simulink model "GPS32"  (R2020b)
settings: Solver=FixedStepAuto  StartTime=0.0  StopTime=inf  FixedStep=0.01  RelTol=1e-3  EnableMultiTasking=on
model workspace (MAT data in the model file):
  Ts = 0.01
values from neighbouring files (symbols this model uses):
  den_lpf_d = den_lpf20    [Mainframe_init.m]    (also in load_autopilot.m)
  num_lpf_d = num_lpf20    [Mainframe_init.m]    (also in load_autopilot.m)
undefined symbols (not defined in the file or in its folder): Autopilot, AUX, dev, DiscIntNeverNeededParam, h_bkpts_m, HIL_Data, Ki_phi_vec, Kp_p_vec, Kp_phi_vec, Main, pwm_output0, pwm_output1, Tr4r3, unc_fin_def_pitch, unc_fin_def_roll, unc_fin_def_yaw, V_bkpts_mps, x, y, z
libraries: simulink_extras x11, px4uORBlib x6, px4Sensorslib x3, px4lib x3, simulink x1, sharedtransform x1
settings Model: SimulationMode=external  ExtModeTrigDuration=10  Creator=WrySi  LastModifiedBy=sasson
settings SolverCC: PositivePriorityOrder=on
settings OptimizationCC: EnhancedBackFolding=on  PassReuseOutputArgsAs=Individual arguments  ZeroExternalMemoryAtStartup=off  ZeroInternalMemoryAtStartup=off  MaxStackSize=64  OptimizeBlockOrder=speed  DifferentSizesBufferReuse=on  OptimizationCustomize=off  EfficientTunableParamExpr=on
settings DebuggingCC: MultiTaskRateTransMsg=warning  ParameterOverflowMsg=none  ParameterTunabilityLossMsg=error  SymbolicDimsDataTypeCodeGenerationDiagnostic=none
settings HardwareCC: ProdBitPerPointer=32  ProdBitPerSizeT=32  ProdBitPerPtrDiffT=32  ProdLargestAtomicInteger=Long  ProdLargestAtomicFloat=Double  ProdWordSize=32  ProdLongLongMode=on  ProdHWDeviceType=ARM Compatible->ARM Cortex
settings SFSimCC: MATLABDynamicMemAlloc=off  SimTargetLang=C++
settings RTWCC: Description=Embedded Coder  SystemTargetFile=ert.tlc  HardwareBoard=PX4 Pixhawk 2.1 (Cube)  TLCOptions="-aInlineSetEventsForThisBaseRateFcn=TLC_FALSE -aSuppressMultiTaskScheduler=TLC_FALSE  -aRateBasedStepFcn=0"  TemplateMakefile=ert_default_tmf  GenerateReport=on  Toolchain=GNU Tools for PX4 Autopilots  IncludeHyperlinkInReport=on  LaunchReport=on  TargetLang=C++  GenerateTraceInfo=on  GenerateTraceReport=on  GenerateTraceReportSl=on  GenerateTraceReportSf=on  GenerateTraceReportEml=on
settings CodeAppCC: ForceParamTrailComments=on  IgnoreCustomStorageClasses=off  OperatorAnnotations=on  SimulinkDataObjDesc=on  SFDataObjDesc=on  InsertBlockDesc=on
settings ERTTargetCC: SupportContinuousTime=on  ExtMode=on  ExtModeMexArgs='127.0.0.1' 1 17725

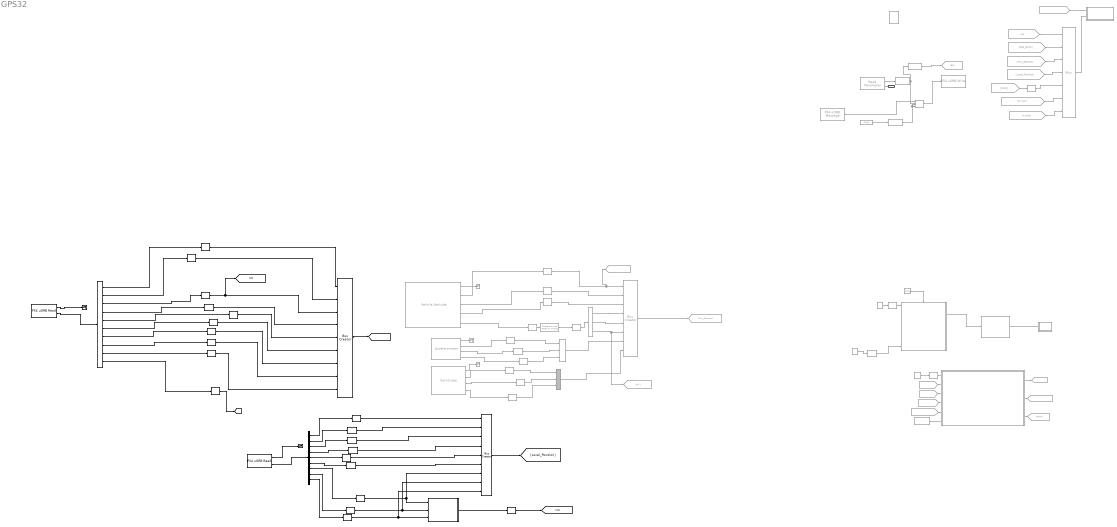
== system GPS32 ==
  note: IMU SENSORS
  note: Debag and Sound
  note: Buzzer
  note: Debag and Sound
  100 Hz : DiscretePulseGenerator  Commented=on  PulseType=Time based  Period=0.01  PulseWidth=50
  Accelerometer : px4Sensorslib/Accelerometer  Commented=on  uorbTimeStamp=off  BlockingMode=off  BlockTimeout=1e-3  sampleTime=Ts
      settings: SourceProductBaseCode=PX4AUTOPILOTS
  Bus Assignment1 : BusAssignment  Commented=on  AssignedSignals=x,z,y
  Bus Creator1 : BusCreator  Inputs=9
  Bus Creator2 : BusCreator  Inputs=9
  Bus Creator6 : BusCreator  Commented=on  Inputs=8
  Bus Creator7 : BusCreator  Commented=on  Inputs=3
  Bus Creator8 : BusCreator  Commented=on  Inputs=3
  Bus Selector1 : BusSelector  OutputSignals=ax,ay,az,z,x,y,vx,vy,vz
  Bus Selector2 : BusSelector  OutputSignals=lat,lon,alt,fix_type,satellites_used,vel_m_s,vel_n_m_s,vel_e_m_s,vel_d_m_s,timestamp
  Cast To Boolean2 : DataTypeConversion  Commented=on  OutDataTypeStr=boolean
  Cast To Double{1,3..9,11,17,21,24..31,33} (20 alike) : DataTypeConversion  OutDataTypeStr=double
  Cast To Double{2,10,12..16,18..20,22..23,32,34..35} (15 alike) : DataTypeConversion  Commented=on  OutDataTypeStr=double
  Constant : Constant  Commented=on  Value=0  SampleTime=Ts
  Constant1 : Constant  Commented=on  Value=0  SampleTime=Ts
  Constant2 : Constant  Commented=on  Value=0  SampleTime=Ts
  Data Type Conversion1 : DataTypeConversion  Commented=on  OutDataTypeStr=single
  Data Type Conversion3 : DataTypeConversion  Commented=on  OutDataTypeStr=single
  Demux2 : Demux  Commented=on  Outputs=3
  Digital Clock2 : DigitalClock  Commented=on
  Fin Allocation : Subsystem  Commented=on
  From : From  Commented=on  GotoTag=Vel
  From1 : From  Commented=on  GotoTag=Alt
  From11 : From  Commented=on  GotoTag=Local_Position
  From14 : From  Commented=on  GotoTag=EN
  From16 : From  Commented=on  GotoTag=Imu_Sensors
  From17 : From  Commented=on  GotoTag=GPS_DATA
  From18 : From  Commented=on  GotoTag=PWM
  From2 : From  Commented=on  GotoTag=P
  From3 : From  Commented=on  GotoTag=Phi
  From4 : From  Commented=on
  From7 : From  Commented=on  GotoTag=P_Filter
  From9 : From  Commented=on  GotoTag=Phi_Con
  Goto10 : Goto  Commented=on  GotoTag=EN
  Goto2 : Goto  Commented=on  GotoTag=P
  Goto3 : Goto  Commented=on  GotoTag=Phi
  Goto5 : Goto  Commented=on  GotoTag=Imu_Sensors
  Goto7 : Goto  Commented=on  GotoTag=PWM
  Goto8 : Goto  Commented=on  GotoTag=P_Filter
  Goto9 : Goto  Commented=on  GotoTag=Phi_Con
  Gyroscope : px4Sensorslib/Gyroscope  Commented=on  uorbTimeStamp=off  BlockingMode=off  BlockTimeout=1e-3  sampleTime=Ts
      settings: SourceProductBaseCode=PX4AUTOPILOTS
  Heartbeat Counter : Subsystem  Commented=on
  MATLAB Function : MATLAB Function  TreatAsAtomicUnit=on
  Mux : Mux  Commented=on  Inputs=7
  PX4 SD Card Logger3 : Subsystem  Commented=on  mask(PX4 SD Card Logger){logfile=/fs/microsd/log, logfilename=pwm, cacheflag=off, numRecs=100000000000000}
      mask prompts: logfile "Log Folder"; logfilename "Log File Name"; cacheflag "Cache in Memory"; numRecs "Maximum Record Count"
      mask help:
      | Log data to a specified file on the SD card
      |
      | The block accepts two inputs, enable and data. The incoming data is logged into the SD card when the enable signal is high and the number of data points logged is less than the Maximum Record Count specified.
      |
      | The specified folder should be present in the SD card for logging.
      |
      | If Cache in Memory is unchecked, the data is written to the SD card at every timestep.  If Cache in Memory is checked, data is cached in the memory and is written to SD card only when enable goes low or when the number of data points logged reaches the Maximum Record Count specified.
      mask init:
      | logname=uint8([logfile,'/',logfilename]);
      mask Help: eval('codertarget.internal.helpView(''px4'',''px4sdcardexample'')');
      mask Display:
      | fprintf([get_param(gcb,'logfile'),'/',get_param(gcb,'logfilename')])
      | port_label('input',1,'en')
      | port_label('input',2,'data')
  PX4 uORB Message : px4uORBlib/PX4 uORB Message  Commented=on  uORBTopic=debug_vect  SampleTime=1  selectInstance=debug_vect
      settings: SourceProductBaseCode=PX4AUTOPILOTS
  PX4 uORB Read1 : px4uORBlib/PX4 uORB Read  uORBTopic=vehicle_local_position  selectInstance=vehicle_local_position  SampleTime=Ts  BlockingMode=off  BlockTimeout=1e-3
      settings: SourceProductBaseCode=PX4AUTOPILOTS
  PX4 uORB Read2 : px4uORBlib/PX4 uORB Read  uORBTopic=vehicle_gps_position  selectInstance=vehicle_gps_position  SampleTime=Ts  BlockingMode=off  BlockTimeout=1e-3
      settings: SourceProductBaseCode=PX4AUTOPILOTS
  PX4 uORB Write : px4uORBlib/PX4 uORB Write  Commented=on  uORBTopic=debug_vect  selectInstance=debug_vect  MessageQueueLen=1
      settings: SourceProductBaseCode=PX4AUTOPILOTS
  Phi Controller : Subsystem  Commented=on
  PixBlock2 : Subsystem  Commented=on
  Quaternions to Rotation Angles2 : sharedtransform/Quaternions to Rotation Angles  Commented=on  rotationOrder=ZYX  aMode=aMode
      settings: SourceProductBaseCode=AE,PW,DR,MT,UV,VE
  Read Parameter1 : px4lib/Read Parameter  Commented=on  ParameterName=SD_save_flag  DataType=INT32  SampleTime=1
      settings: SourceProductBaseCode=PX4AUTOPILOTS
  Servos : Subsystem  Commented=on
  Subsystem2 : Subsystem  Commented=on
  Terminator1 : Terminator
  Terminator3 : Terminator
  Terminator7 : Terminator  Commented=on
  Terminator8 : Terminator  Commented=on
  Terminator9 : Terminator  Commented=on
  Vehicle Attitude : px4Sensorslib/Vehicle Attitude  Commented=on  rollRate=on  pitchRate=on  yawRate=on  quaternion=on  uorbTimeStamp=off  BlockingMode=off  BlockTimeout=0.001  sampleTime=Ts
      settings: SourceProductBaseCode=PX4AUTOPILOTS
  Out1 : Outport
  wires:
  Bus Selector2/9 -> Cast To Double11/1  "<vel_d_m_s>"
  Bus Selector2/6 -> Cast To Double7/1  "<vel_m_s>"
  Gyroscope/4 -> Cast To Double18/1  "gyroZ"
  Accelerometer/4 -> Cast To Double10/1  "accZ"
  Accelerometer/1 -> Terminator7/1
  Cast To Double2/1 -> Quaternions to Rotation Angles2/1
  Gyroscope/3 -> Cast To Double19/1  "gyroY"
  Vehicle Attitude/5 -> Cast To Double2/1
  Bus Creator7/1 -> Bus Creator6/7  "accelerometer"
  Gyroscope/1 -> Terminator9/1
  Gyroscope/2 -> Cast To Double20/1  "gyroX"
  Bus Selector2/3 -> Cast To Double4/1  "<alt>"
  Accelerometer/3 -> Cast To Double12/1  "accY"
  Accelerometer/2 -> Cast To Double13/1  "accX"
  Bus Creator8/1 -> Bus Creator6/8  "gyro"
  Vehicle Attitude/2 -> Cast To Double16/1  "p"
  Vehicle Attitude/3 -> Cast To Double15/1  "q"
  Quaternions to Rotation Angles2/1 -> Cast To Double22/1  "euler from PX conj"
  Vehicle Attitude/4 -> Cast To Double14/1  "r"
  Bus Selector2/7 -> Cast To Double8/1  "<vel_n_m_s>"
  PX4 uORB Read2/2 -> Bus Selector2/1
  Bus Selector2/8 -> Cast To Double9/1  "<vel_e_m_s>"
  Bus Selector2/1 -> Cast To Double1/1  "<lat>"
  Bus Selector2/4 -> Cast To Double5/1  "<fix_type>"
  Bus Selector2/5 -> Cast To Double6/1  "<satellites_used>"
  Vehicle Attitude/1 -> Terminator8/1
  Bus Selector2/2 -> Cast To Double3/1  "<lon>"
  Cast To Double1/1 -> Bus Creator2/1
  Cast To Double3/1 -> Bus Creator2/2
  Cast To Double4/1 -> Bus Creator2/3, [Alt]
  Cast To Double5/1 -> Bus Creator2/4
  Cast To Double6/1 -> Bus Creator2/5
  Cast To Double7/1 -> Bus Creator2/6
  Cast To Double8/1 -> Bus Creator2/7
  Cast To Double9/1 -> Bus Creator2/8
  Cast To Double11/1 -> Bus Creator2/9
  Cast To Double16/1 -> Bus Creator6/1, Goto2/1
  Cast To Double15/1 -> Bus Creator6/2
  Cast To Double14/1 -> Bus Creator6/3
  Cast To Double12/1 -> Bus Creator7/2
  Cast To Double10/1 -> Bus Creator7/3
  Cast To Double13/1 -> Bus Creator7/1
  Cast To Double20/1 -> Bus Creator8/1
  Cast To Double19/1 -> Bus Creator8/2
  Cast To Double18/1 -> Bus Creator8/3
  PX4 uORB Read2/1 -> Terminator1/1
  PX4 uORB Read1/2 -> Bus Selector1/1
  Bus Selector1/1 -> Cast To Double17/1  "<ax>"
  Bus Selector1/2 -> Cast To Double24/1  "<ay>"
  PX4 uORB Read1/1 -> Terminator3/1
  Bus Selector1/3 -> Cast To Double25/1  "<az>"
  Bus Selector1/4 -> Cast To Double26/1  "<z>"
  Bus Selector1/5 -> Cast To Double27/1  "<x>"
  Bus Selector1/6 -> Cast To Double28/1  "<y>"
  Cast To Double22/1 -> Demux2/1
  Cast To Double26/1 -> Bus Creator1/4
  Cast To Double27/1 -> Bus Creator1/5
  Cast To Double28/1 -> Bus Creator1/6
  Cast To Double25/1 -> Bus Creator1/3
  Cast To Double24/1 -> Bus Creator1/2
  Bus Assignment1/1 -> PX4 uORB Write/1
  Data Type Conversion1/1 -> Bus Assignment1/3, Bus Assignment1/4
  PX4 uORB Message/1 -> Bus Assignment1/1
  Read Parameter1/1 -> Data Type Conversion3/1
  Read Parameter1/2 -> Out1/1
  Digital Clock2/1 -> Data Type Conversion1/1
  Data Type Conversion3/1 -> Bus Assignment1/2, Cast To Boolean2/1
  Cast To Double29/1 -> Bus Creator1/7, MATLAB Function/1(vx)
  Cast To Double31/1 -> Bus Creator1/9, MATLAB Function/3(vz)
  Bus Selector1/8 -> Cast To Double30/1  "<vy>"
  Cast To Double30/1 -> Bus Creator1/8, MATLAB Function/2(vy)
  Bus Selector1/7 -> Cast To Double29/1  "<vx>"
  Bus Selector1/9 -> Cast To Double31/1  "<vz>"
  MATLAB Function/1(y) -> Cast To Double33/1
  Cast To Double23/1 -> Phi Controller/1(phi_cmd_rad)
  Constant/1 -> Cast To Double23/1
  Demux2/3 -> Goto3/1, Bus Creator6/6  "phi"
  Demux2/2 -> Bus Creator6/5  "theta"
  Demux2/1 -> Bus Creator6/4  "psi"
  Bus Creator6/1 -> Goto5/1
  Bus Creator1/1 -> [Local_Position]
  Cast To Double17/1 -> Bus Creator1/1
  Bus Creator2/1 -> [GPS_DATA]
  Cast To Double33/1 -> [Vel]
  Cast To Boolean2/1 -> Goto10/1
  From14/1 -> PX4 SD Card Logger3/1(En)
  Bus Selector2/10 -> Cast To Double21/1  "<timestamp>"
  Cast To Double21/1 -> [A]
  100 Hz/1 -> Phi Controller/Trigger
  Constant1/1 -> Cast To Double32/1
  Phi Controller/1(dela_cmd_rad) -> Fin Allocation/1(Input)  "Phi_Cmd_rad"
  Fin Allocation/1(siB_cmd) -> Servos/1(Fin Cmd)
  Cast To Double32/1 -> Phi Controller/6(integrators_active)
  From17/1 -> Mux/2
  From16/1 -> Mux/3
  From11/1 -> Mux/4
  From9/1 -> Mux/6
  From7/1 -> Mux/7
  Mux/1 -> PX4 SD Card Logger3/2(Data)
  From18/1 -> Cast To Double35/1
  Cast To Double35/1 -> Mux/5
  From4/1 -> Mux/1
  Heartbeat Counter/1(Out1) -> PixBlock2/6(Heartbeat)  "send"
  Cast To Double34/1 -> PixBlock2/1(Phi_cmd)
  Constant2/1 -> Cast To Double34/1
  From2/1 -> PixBlock2/2(P_rms)
  From1/1 -> PixBlock2/3(Alt)
  From/1 -> PixBlock2/4(Velocity)
  From3/1 -> PixBlock2/5(Phi)
  PixBlock2/2(Fin_cmd) -> Goto9/1
  PixBlock2/3(PWM) -> Goto7/1
  PixBlock2/1(P_filter) -> Goto8/1

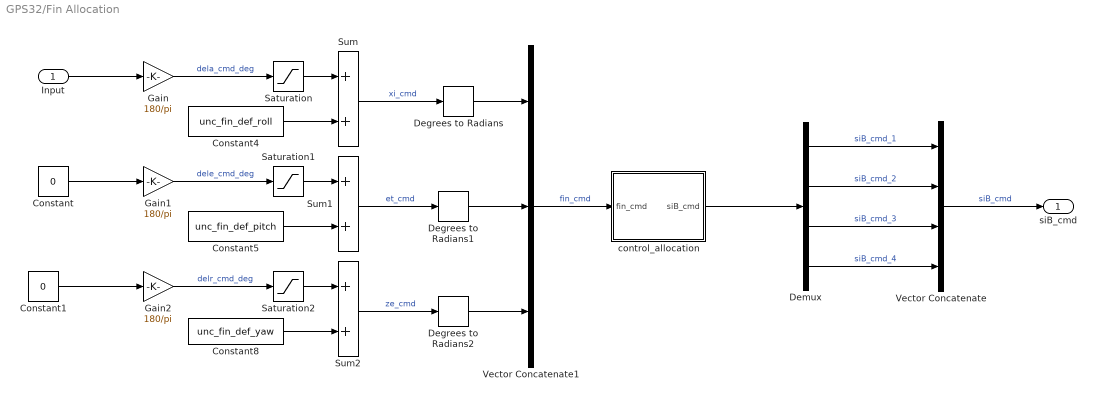
== system GPS32/Fin Allocation ==
  Input : Inport
  Constant : Constant  Value=0
  Constant1 : Constant  Value=0
  Constant4 : Constant  Value=unc_fin_def_roll
  Constant5 : Constant  Value=unc_fin_def_pitch
  Constant8 : Constant  Value=unc_fin_def_yaw
  Degrees to Radians : simulink_extras/Transformations/Degrees to Radians
  Degrees to Radians1 : simulink_extras/Transformations/Degrees to Radians
  Degrees to Radians2 : simulink_extras/Transformations/Degrees to Radians
  Demux : Demux
  Gain : Gain  Gain=180/pi
      settings: AttributesFormatString=%<Gain>
  Gain1 : Gain  Gain=180/pi
      settings: AttributesFormatString=%<Gain>
  Gain2 : Gain  Gain=180/pi
      settings: AttributesFormatString=%<Gain>
  Saturation : Saturate  UpperLimit=20  LowerLimit=-20
  Saturation1 : Saturate  UpperLimit=20  LowerLimit=-20
  Saturation2 : Saturate  UpperLimit=20  LowerLimit=-20
  Sum : Sum
  Sum1 : Sum
  Sum2 : Sum
  Vector Concatenate : Concatenate  NumInputs=4
  Vector Concatenate1 : Concatenate  NumInputs=3
  control_allocation : Subsystem
  siB_cmd : Outport  VectorParamsAs1DForOutWhenUnconnected=off
  wires:
  Constant5/1 -> Sum1/2
  Gain2/1 -> Saturation2/1  "delr_cmd_deg"
  Saturation2/1 -> Sum2/1
  Constant8/1 -> Sum2/2
  Sum2/1 -> Degrees to Radians2/1  "ze_cmd"
  Demux/3 -> Vector Concatenate/3  "siB_cmd_3"
  Constant1/1 -> Gain2/1
  Saturation/1 -> Sum/1
  Gain1/1 -> Saturation1/1  "dele_cmd_deg"
  Sum1/1 -> Degrees to Radians1/1  "et_cmd"
  Degrees to Radians/1 -> Vector Concatenate1/1
  Degrees to Radians1/1 -> Vector Concatenate1/2
  Gain/1 -> Saturation/1  "dela_cmd_deg"
  Input/1 -> Gain/1
  Degrees to Radians2/1 -> Vector Concatenate1/3
  Demux/2 -> Vector Concatenate/2  "siB_cmd_2"
  Constant4/1 -> Sum/2
  Vector Concatenate/1 -> siB_cmd/1  "siB_cmd"
  Constant/1 -> Gain1/1
  Sum/1 -> Degrees to Radians/1  "xi_cmd"
  Saturation1/1 -> Sum1/1
  Vector Concatenate1/1 -> control_allocation/1(fin_cmd)  "fin_cmd"
  Demux/1 -> Vector Concatenate/1  "siB_cmd_1"
  control_allocation/1(siB_cmd) -> Demux/1
  Demux/4 -> Vector Concatenate/4  "siB_cmd_4"

== system GPS32/Heartbeat Counter ==
  note: Starting the heartbeat at negative values prevents unwanted FCC behaviour on startup
  Cast To Double14 : DataTypeConversion  OutDataTypeStr=single
  Heartbeat : simulink/Sources/Counter Free-Running  NumBits=16  tsamp=-1
  Subtract : Sum  Inputs=+-
  Zero : Constant  Value=1000  OutDataTypeStr=Inherit: Inherit via back propagation
  Out1 : Outport
  wires:
  Heartbeat/1 -> Cast To Double14/1
  Zero/1 -> Subtract/2
  Cast To Double14/1 -> Subtract/1  "send"
  Subtract/1 -> Out1/1

== system GPS32/PX4 SD Card Logger3 ==
  En : Inport
  Data : Inport  Port=2
  SDCard_logger : MATLAB Function  TreatAsAtomicUnit=on
  Signal Specification : SignalSpecification  OutDataTypeStr=boolean
  wires:
  Data/1 -> SDCard_logger/2(data)
  En/1 -> Signal Specification/1
  Signal Specification/1 -> SDCard_logger/1(en)

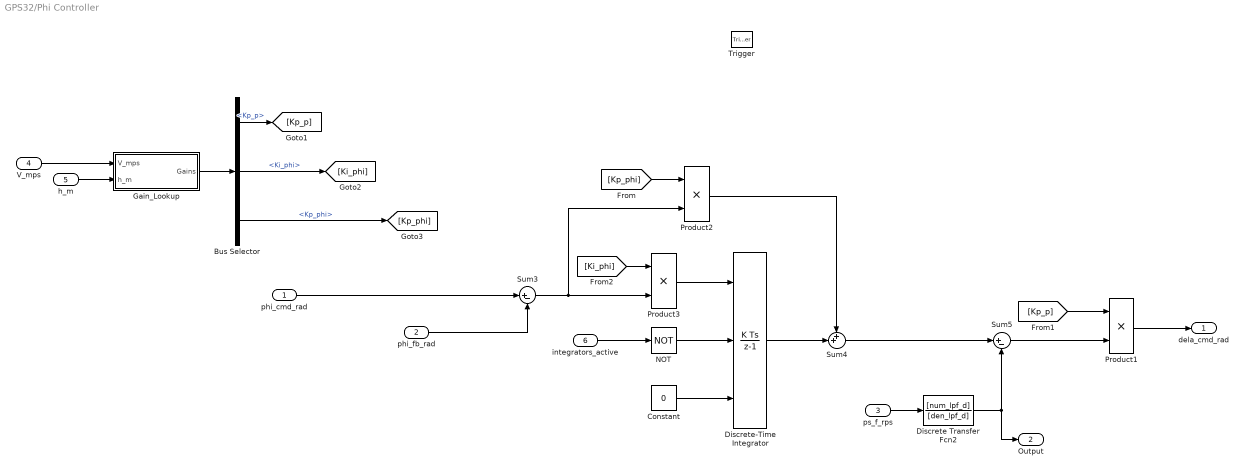
== system GPS32/Phi Controller ==
  phi_cmd_rad : Inport
  phi_fb_rad : Inport  Port=2
  ps_f_rps : Inport  Port=3
  V_mps : Inport  Port=4
  h_m : Inport  Port=5
  integrators_active : Inport  Port=6
  Trigger : TriggerPort  VariantControl=Variant  PortDimensions=1
  Bus Selector : BusSelector  OutputSignals=Kp_p,Ki_phi,Kp_phi
  Constant : Constant  Value=0  SampleTime=-1
  Discrete Transfer Fcn2 : DiscreteTransferFcn  Numerator=[num_lpf_d]  Denominator=[den_lpf_d]
  Discrete-Time Integrator : DiscreteIntegrator  ExternalReset=level  InitialConditionSource=external  SampleTime=-1  ICPrevOutput=DiscIntNeverNeededParam  ICPrevScaledInput=DiscIntNeverNeededParam
  Gain_Lookup : Subsystem
  NOT : Logic  Operator=NOT  AllPortsSameDT=off  OutDataTypeStr=boolean
  Product1 : Product
  Product2 : Product
  Product3 : Product
  Sum3 : Sum  Inputs=|+-
  Sum4 : Sum  Inputs=++|
  Sum5 : Sum  Inputs=|+-
  dela_cmd_rad : Outport
  Output : Outport  Port=2
  wires:
  Discrete-Time Integrator/1 -> Sum4/2
  NOT/1 -> Discrete-Time Integrator/2
  Bus Selector/2 -> [Ki_phi]  "<Ki_phi>"
  Product1/1 -> dela_cmd_rad/1
  ps_f_rps/1 -> Discrete Transfer Fcn2/1
  [Kp_phi] -> Product2/1
  h_m/1 -> Gain_Lookup/2(h_m)
  V_mps/1 -> Gain_Lookup/1(V_mps)
  integrators_active/1 -> NOT/1
  Constant/1 -> Discrete-Time Integrator/3
  [Kp_p] -> Product1/1
  Sum5/1 -> Product1/2
  phi_cmd_rad/1 -> Sum3/1
  Sum4/1 -> Sum5/1
  Gain_Lookup/1(Gains) -> Bus Selector/1
  Product3/1 -> Discrete-Time Integrator/1
  Bus Selector/1 -> [Kp_p]  "<Kp_p>"
  phi_fb_rad/1 -> Sum3/2
  Bus Selector/3 -> [Kp_phi]  "<Kp_phi>"
  [Ki_phi] -> Product3/1
  Product2/1 -> Sum4/1
  Sum3/1 -> Product3/2, Product2/2
  Discrete Transfer Fcn2/1 -> Output/1, Sum5/2

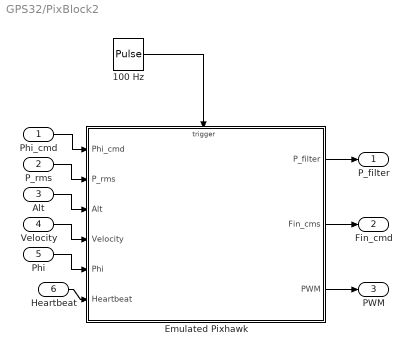
== system GPS32/PixBlock2 ==
  Phi_cmd : Inport
  P_rms : Inport  Port=2
  Alt : Inport  Port=3
  Velocity : Inport  Port=4
  Phi : Inport  Port=5
  Heartbeat : Inport  Port=6
  100 Hz : DiscretePulseGenerator  PulseType=Time based  Period=0.01  PulseWidth=50
  Emulated Pixhawk : Subsystem
  P_filter : Outport
  Fin_cmd : Outport  Port=2
  PWM : Outport  Port=3
  wires:
  100 Hz/1 -> Emulated Pixhawk/Trigger
  Emulated Pixhawk/1(P_filter) -> P_filter/1
  Phi_cmd/1 -> Emulated Pixhawk/1(Phi_cmd)
  P_rms/1 -> Emulated Pixhawk/2(P_rms)
  Phi/1 -> Emulated Pixhawk/5(Phi)
  Velocity/1 -> Emulated Pixhawk/4(Velocity)
  Alt/1 -> Emulated Pixhawk/3(Alt)
  Emulated Pixhawk/2(Fin_cms) -> Fin_cmd/1
  Heartbeat/1 -> Emulated Pixhawk/6(Heartbeat)
  Emulated Pixhawk/3(PWM) -> PWM/1

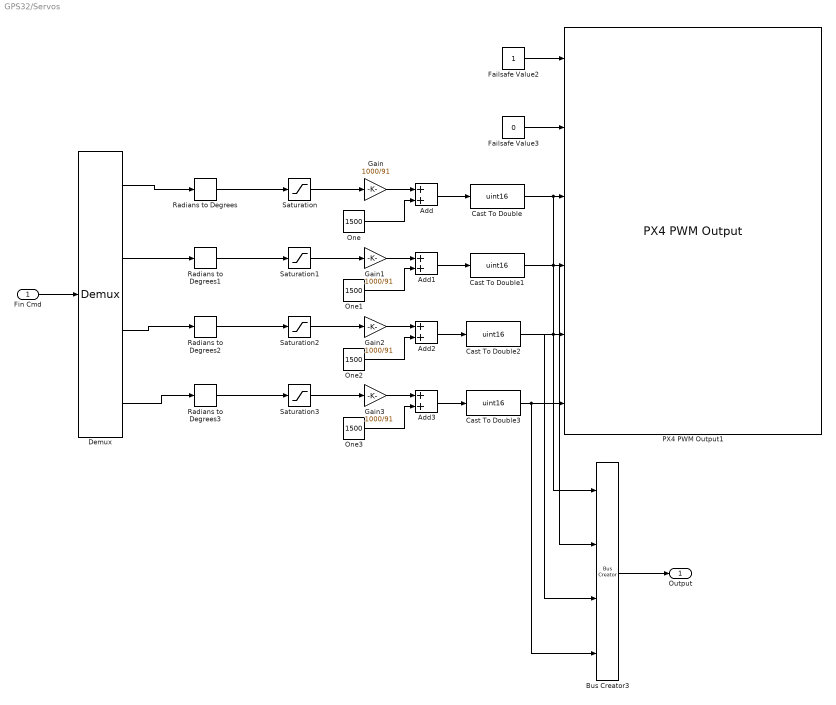
== system GPS32/Servos ==
  Fin Cmd : Inport
  Add{,1..3} (4 alike) : Sum
  Bus Creator3 : BusCreator  Inputs=4
  Cast To Double{,1..3} (4 alike) : DataTypeConversion  OutDataTypeStr=uint16
  Demux : Demux
  Failsafe Value2 : Constant  OutDataTypeStr=boolean  SampleTime=-1
  Failsafe Value3 : Constant  Value=0  OutDataTypeStr=boolean  SampleTime=-1
  Gain{,1..3} (4 alike) : Gain  Gain=1000/91
  One{,1..3} (4 alike) : Constant  Value=1500  OutDataTypeStr=Inherit: Inherit via back propagation
  PX4 PWM Output1 : px4lib/PX4 PWM Output  pwmDevice=Main (/dev/pwm_output0)  pwmChannel1_=on  pwmChannel2_=on  pwmChannel3_=on  pwmChannel4_=on  pwmChannel5_=off  pwmChannel6_=off  pwmChannel7_=off  pwmChannel8_=off  forceTerminateFailsafe=off  outputErrorStatus=off
      settings: SourceProductBaseCode=PX4AUTOPILOTS
  Radians to Degrees{,1..3} (4 alike) : simulink_extras/Transformations/Radians to Degrees
  Saturation{,1..3} (4 alike) : Saturate  UpperLimit=20  LowerLimit=-20
  Output : Outport
  wires:
  Saturation2/1 -> Gain2/1
  Cast To Double3/1 -> Bus Creator3/4, PX4 PWM Output1/6
  Failsafe Value3/1 -> PX4 PWM Output1/2
  One/1 -> Add/2
  One2/1 -> Add2/2
  Add1/1 -> Cast To Double1/1
  Gain2/1 -> Add2/1
  Radians to Degrees1/1 -> Saturation1/1
  Cast To Double2/1 -> Bus Creator3/3, PX4 PWM Output1/5
  Add2/1 -> Cast To Double2/1
  Cast To Double1/1 -> Bus Creator3/2, PX4 PWM Output1/4
  Gain/1 -> Add/1
  Demux/4 -> Radians to Degrees3/1
  One3/1 -> Add3/2
  Saturation/1 -> Gain/1
  Gain1/1 -> Add1/1
  Saturation3/1 -> Gain3/1
  Gain3/1 -> Add3/1
  Radians to Degrees3/1 -> Saturation3/1
  Demux/1 -> Radians to Degrees/1
  Demux/3 -> Radians to Degrees2/1
  Saturation1/1 -> Gain1/1
  Cast To Double/1 -> Bus Creator3/1, PX4 PWM Output1/3
  Add3/1 -> Cast To Double3/1
  Radians to Degrees2/1 -> Saturation2/1
  Radians to Degrees/1 -> Saturation/1
  One1/1 -> Add1/2
  Add/1 -> Cast To Double/1
  Failsafe Value2/1 -> PX4 PWM Output1/1
  Bus Creator3/1 -> Output/1
  Demux/2 -> Radians to Degrees1/1
  Fin Cmd/1 -> Demux/1

== system GPS32/Subsystem2 ==
  Bus Assignment : BusAssignment  AssignedSignals=tune_id
  Constant : Constant  Value=2  OutDataTypeStr=uint8  SampleTime=60
  PX4 uORB Message1 : px4uORBlib/PX4 uORB Message  uORBTopic=tune_control  SampleTime=60  selectInstance=tune_control
      settings: SourceProductBaseCode=PX4AUTOPILOTS
  PX4 uORB Write1 : px4uORBlib/PX4 uORB Write  uORBTopic=tune_control  selectInstance=tune_control  MessageQueueLen=1
      settings: SourceProductBaseCode=PX4AUTOPILOTS
  wires:
  PX4 uORB Message1/1 -> Bus Assignment/1
  Bus Assignment/1 -> PX4 uORB Write1/1
  Constant/1 -> Bus Assignment/2

== system GPS32/Fin Allocation/control_allocation ==
  fin_cmd : Inport
  Constant7 : Constant  Value=Tr4r3
  Product : Product  Multiplication=Matrix(*)
  siB_cmd : Outport  VectorParamsAs1DForOutWhenUnconnected=off
  wires:
  Constant7/1 -> Product/1
  fin_cmd/1 -> Product/2
  Product/1 -> siB_cmd/1  "siB_cmd"

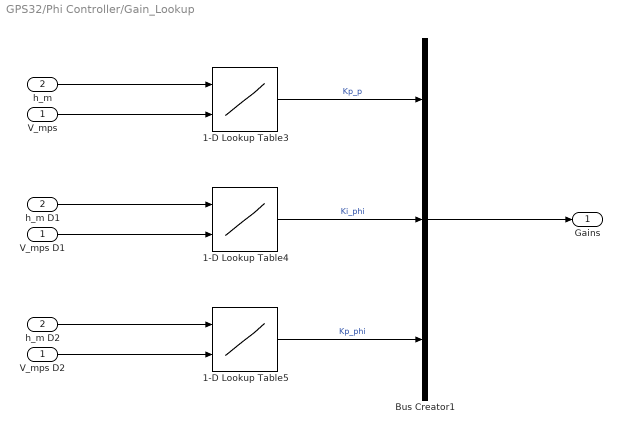
== system GPS32/Phi Controller/Gain_Lookup ==
  V_mps : Inport
  h_m : Inport  Port=2
  1-D Lookup Table3 : Lookup_n-D  BreakpointsForDimension1=h_bkpts_m  BreakpointsForDimension2=V_bkpts_mps  Table=Kp_p_vec  ExtrapMethod=Clip  UseLastTableValue=on  InternalRulePriority=Speed  RndMeth=Simplest  InputSameDT=on
      settings: InputPortMap=u0,u1
      settings: AttributesFormatString=|
      | %<Table>
      | %<BreakpointsForDimension1>
      | %<BreakpointsForDimension2>
  1-D Lookup Table4 : Lookup_n-D  BreakpointsForDimension1=h_bkpts_m  BreakpointsForDimension2=V_bkpts_mps  Table=Ki_phi_vec  ExtrapMethod=Clip  UseLastTableValue=on  InternalRulePriority=Speed  RndMeth=Simplest  InputSameDT=on
      settings: InputPortMap=u0,u1
      settings: AttributesFormatString=|
      | %<Table>
      | %<BreakpointsForDimension1>
      | %<BreakpointsForDimension2>
  1-D Lookup Table5 : Lookup_n-D  BreakpointsForDimension1=h_bkpts_m  BreakpointsForDimension2=V_bkpts_mps  Table=Kp_phi_vec  ExtrapMethod=Clip  UseLastTableValue=on  InternalRulePriority=Speed  RndMeth=Simplest  InputSameDT=on
      settings: InputPortMap=u0,u1
      settings: AttributesFormatString=|
      | %<Table>
      | %<BreakpointsForDimension1>
      | %<BreakpointsForDimension2>
  Bus Creator1 : BusCreator  Inputs=3
  V_mps D1 : InportShadow
  V_mps D2 : InportShadow
  h_m D1 : InportShadow  Port=2
  h_m D2 : InportShadow  Port=2
  Gains : Outport
  wires:
  h_m/1 -> 1-D Lookup Table3/1
  Bus Creator1/1 -> Gains/1
  1-D Lookup Table5/1 -> Bus Creator1/3  "Kp_phi"
  1-D Lookup Table4/1 -> Bus Creator1/2  "Ki_phi"
  1-D Lookup Table3/1 -> Bus Creator1/1  "Kp_p"
  V_mps/1 -> 1-D Lookup Table3/2
  h_m D1/1 -> 1-D Lookup Table4/1
  V_mps D1/1 -> 1-D Lookup Table4/2
  h_m D2/1 -> 1-D Lookup Table5/1
  V_mps D2/1 -> 1-D Lookup Table5/2

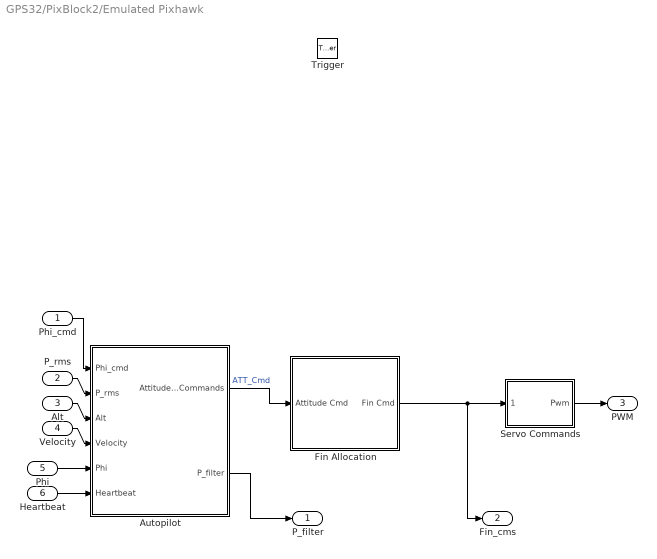
== system GPS32/PixBlock2/Emulated Pixhawk ==
  Phi_cmd : Inport
  P_rms : Inport  Port=2
  Alt : Inport  Port=3
  Velocity : Inport  Port=4
  Phi : Inport  Port=5
  Heartbeat : Inport  Port=6
  Trigger : TriggerPort  VariantControl=Variant  PortDimensions=1
  Autopilot : Subsystem
  Fin Allocation : Subsystem
  Servo Commands : Subsystem
  P_filter : Outport  VectorParamsAs1DForOutWhenUnconnected=off
  Fin_cms : Outport  Port=2  VectorParamsAs1DForOutWhenUnconnected=off
  PWM : Outport  Port=3  VectorParamsAs1DForOutWhenUnconnected=off
  wires:
  Alt/1 -> Autopilot/3(Alt)
  Fin Allocation/1(Fin Cmd) -> Fin_cms/1, Servo Commands/1(Fin Cmd)
  Autopilot/1(Attitude_Commands) -> Fin Allocation/1(Attitude Cmd)  "ATT_Cmd"
  Phi_cmd/1 -> Autopilot/1(Phi_cmd)
  Velocity/1 -> Autopilot/4(Velocity)
  Phi/1 -> Autopilot/5(Phi)
  P_rms/1 -> Autopilot/2(P_rms)
  Autopilot/2(P_filter) -> P_filter/1
  Heartbeat/1 -> Autopilot/6(Heartbeat)
  Servo Commands/1(Pwm) -> PWM/1

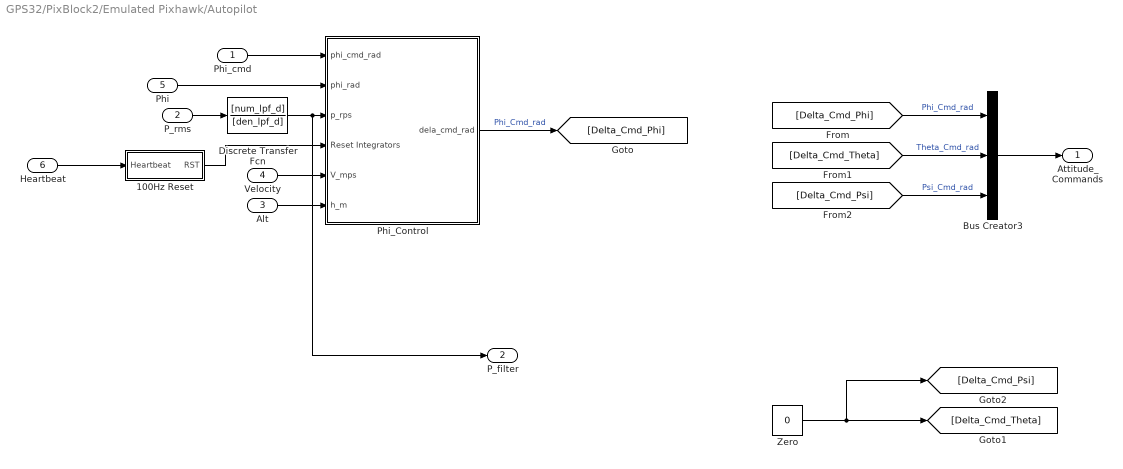
== system GPS32/PixBlock2/Emulated Pixhawk/Autopilot ==
  Phi_cmd : Inport
  P_rms : Inport  Port=2
  Alt : Inport  Port=3
  Velocity : Inport  Port=4
  Phi : Inport  Port=5
  Heartbeat : Inport  Port=6
  100Hz Reset : Subsystem
  Bus Creator3 : BusCreator  Inputs=3
  Discrete Transfer Fcn : DiscreteTransferFcn  Numerator=[num_lpf_d]  Denominator=[den_lpf_d]
  Phi_Control : Subsystem
  Zero : Constant  Value=0  OutDataTypeStr=Inherit: Inherit via back propagation
  Attitude_Commands : Outport  VectorParamsAs1DForOutWhenUnconnected=off
  P_filter : Outport  Port=2  VectorParamsAs1DForOutWhenUnconnected=off
  wires:
  P_rms/1 -> Discrete Transfer Fcn/1
  Velocity/1 -> Phi_Control/5(V_mps)
  Zero/1 -> [Delta_Cmd_Psi], [Delta_Cmd_Theta]
  [Delta_Cmd_Phi] -> Bus Creator3/1  "Phi_Cmd_rad"
  [Delta_Cmd_Theta] -> Bus Creator3/2  "Theta_Cmd_rad"
  Bus Creator3/1 -> Attitude_Commands/1
  [Delta_Cmd_Psi] -> Bus Creator3/3  "Psi_Cmd_rad"
  100Hz Reset/1(RST) -> Phi_Control/4(Reset Integrators)
  Alt/1 -> Phi_Control/6(h_m)
  Phi_Control/1(dela_cmd_rad) -> [Delta_Cmd_Phi]  "Phi_Cmd_rad"
  Discrete Transfer Fcn/1 -> P_filter/1, Phi_Control/3(p_rps)
  Phi/1 -> Phi_Control/2(phi_rad)
  Heartbeat/1 -> 100Hz Reset/1(Heartbeat)
  Phi_cmd/1 -> Phi_Control/1(phi_cmd_rad)

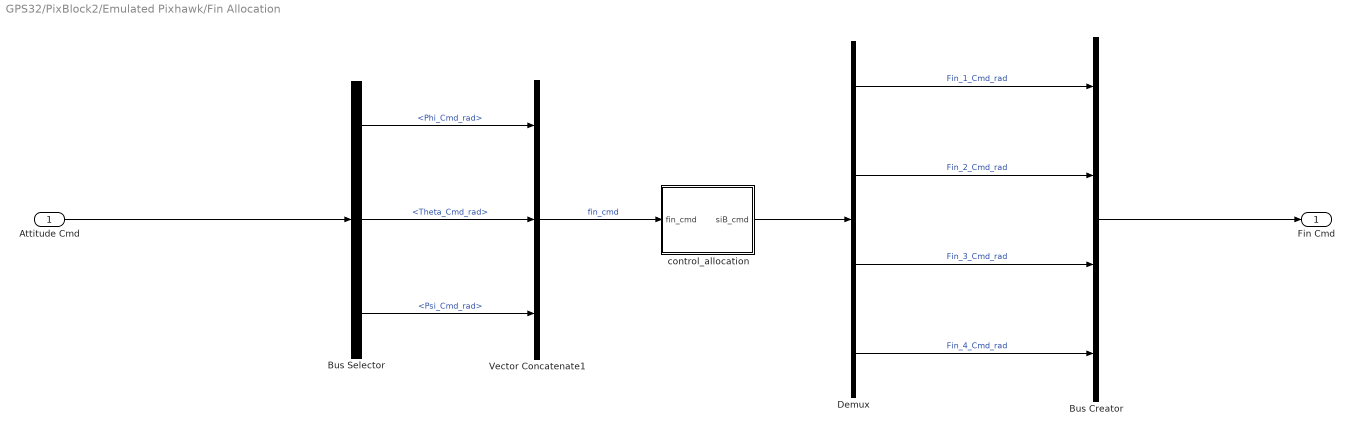
== system GPS32/PixBlock2/Emulated Pixhawk/Fin Allocation ==
  Attitude Cmd : Inport
  Bus Creator : BusCreator  Inputs=4
  Bus Selector : BusSelector  OutputSignals=Phi_Cmd_rad,Theta_Cmd_rad,Psi_Cmd_rad
  Demux : Demux
  Vector Concatenate1 : Concatenate  NumInputs=3
  control_allocation : Subsystem
  Fin Cmd : Outport  VectorParamsAs1DForOutWhenUnconnected=off
  wires:
  Demux/4 -> Bus Creator/4  "Fin_4_Cmd_rad"
  control_allocation/1(siB_cmd) -> Demux/1
  Bus Selector/3 -> Vector Concatenate1/3  "<Psi_Cmd_rad>"
  Vector Concatenate1/1 -> control_allocation/1(fin_cmd)  "fin_cmd"
  Bus Selector/1 -> Vector Concatenate1/1  "<Phi_Cmd_rad>"
  Demux/3 -> Bus Creator/3  "Fin_3_Cmd_rad"
  Bus Selector/2 -> Vector Concatenate1/2  "<Theta_Cmd_rad>"
  Demux/1 -> Bus Creator/1  "Fin_1_Cmd_rad"
  Bus Creator/1 -> Fin Cmd/1
  Attitude Cmd/1 -> Bus Selector/1
  Demux/2 -> Bus Creator/2  "Fin_2_Cmd_rad"

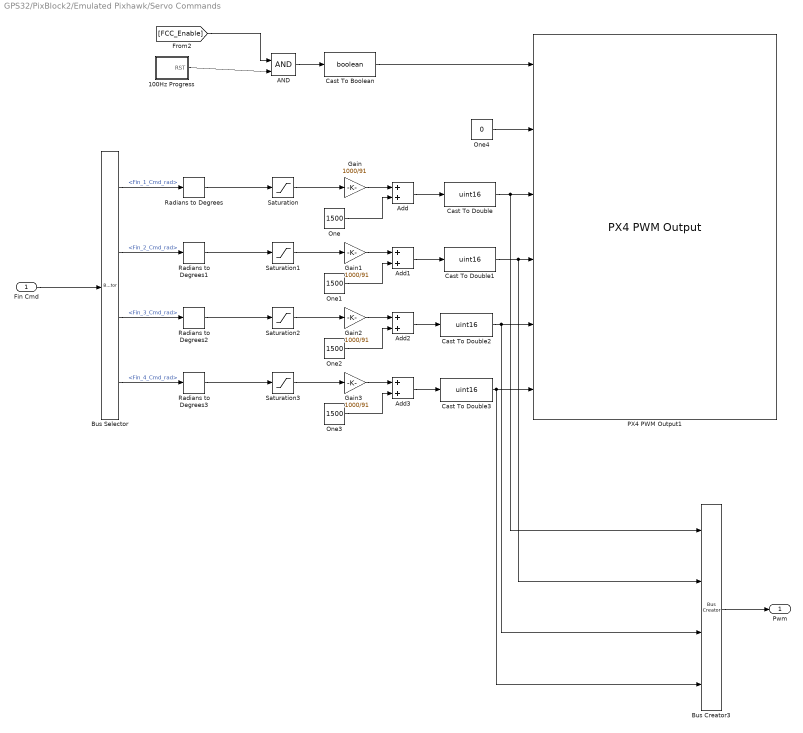
== system GPS32/PixBlock2/Emulated Pixhawk/Servo Commands ==
  Fin Cmd : Inport
  100Hz Progress : Subsystem
  AND : Logic  IconShape=distinctive  AllPortsSameDT=off  OutDataTypeStr=boolean
  Add{,1..3} (4 alike) : Sum
  Bus Creator3 : BusCreator  Inputs=4
  Bus Selector : BusSelector  OutputSignals=Fin_1_Cmd_rad,Fin_2_Cmd_rad,Fin_3_Cmd_rad,Fin_4_Cmd_rad
  Cast To Boolean : DataTypeConversion  OutDataTypeStr=boolean
  Cast To Double{,1..3} (4 alike) : DataTypeConversion  OutDataTypeStr=uint16
  Gain{,1..3} (4 alike) : Gain  Gain=1000/91
  One{,1..3} (4 alike) : Constant  Value=1500  OutDataTypeStr=Inherit: Inherit via back propagation
  One4 : Constant  Value=0  OutDataTypeStr=boolean
  PX4 PWM Output1 : px4lib/PX4 PWM Output  pwmDevice=AUX (/dev/pwm_output1)  pwmChannel1_=on  pwmChannel2_=on  pwmChannel3_=on  pwmChannel4_=on  pwmChannel5_=off  pwmChannel6_=off  pwmChannel7_=off  pwmChannel8_=off  forceTerminateFailsafe=off  outputErrorStatus=off
      settings: SourceProductBaseCode=PX4AUTOPILOTS
  Radians to Degrees{,1..3} (4 alike) : simulink_extras/Transformations/Radians to Degrees
  Saturation{,1..3} (4 alike) : Saturate  UpperLimit=20  LowerLimit=-20
  Pwm : Outport
  wires:
  Saturation2/1 -> Gain2/1
  One4/1 -> PX4 PWM Output1/2
  One/1 -> Add/2
  One2/1 -> Add2/2
  Add1/1 -> Cast To Double1/1
  Gain2/1 -> Add2/1
  AND/1 -> Cast To Boolean/1
  Radians to Degrees1/1 -> Saturation1/1
  Add2/1 -> Cast To Double2/1
  Fin Cmd/1 -> Bus Selector/1
  Bus Selector/2 -> Radians to Degrees1/1  "<Fin_2_Cmd_rad>"
  Gain/1 -> Add/1
  Bus Selector/4 -> Radians to Degrees3/1  "<Fin_4_Cmd_rad>"
  One3/1 -> Add3/2
  Saturation/1 -> Gain/1
  Gain1/1 -> Add1/1
  Saturation3/1 -> Gain3/1
  Gain3/1 -> Add3/1
  Radians to Degrees3/1 -> Saturation3/1
  Bus Selector/1 -> Radians to Degrees/1  "<Fin_1_Cmd_rad>"
  Bus Selector/3 -> Radians to Degrees2/1  "<Fin_3_Cmd_rad>"
  Saturation1/1 -> Gain1/1
  Add3/1 -> Cast To Double3/1
  Radians to Degrees2/1 -> Saturation2/1
  [FCC_Enable] -> AND/1
  Radians to Degrees/1 -> Saturation/1
  100Hz Progress/1(RST) -> AND/2
  One1/1 -> Add1/2
  Add/1 -> Cast To Double/1
  Cast To Boolean/1 -> PX4 PWM Output1/1
  Bus Creator3/1 -> Pwm/1
  Cast To Double/1 -> Bus Creator3/1, PX4 PWM Output1/3
  Cast To Double1/1 -> Bus Creator3/2, PX4 PWM Output1/4
  Cast To Double2/1 -> Bus Creator3/3, PX4 PWM Output1/5
  Cast To Double3/1 -> Bus Creator3/4, PX4 PWM Output1/6

== system GPS32/PixBlock2/Emulated Pixhawk/Autopilot/100Hz Reset ==
  Heartbeat : Inport
  Delay : Delay  DelayLength=1
  GreaterThan : RelationalOperator  Operator=<  OutDataTypeStr=boolean  RndMeth=Simplest
  RST : Outport
  wires:
  GreaterThan/1 -> RST/1
  Delay/1 -> GreaterThan/2
  Heartbeat/1 -> Delay/1, GreaterThan/1

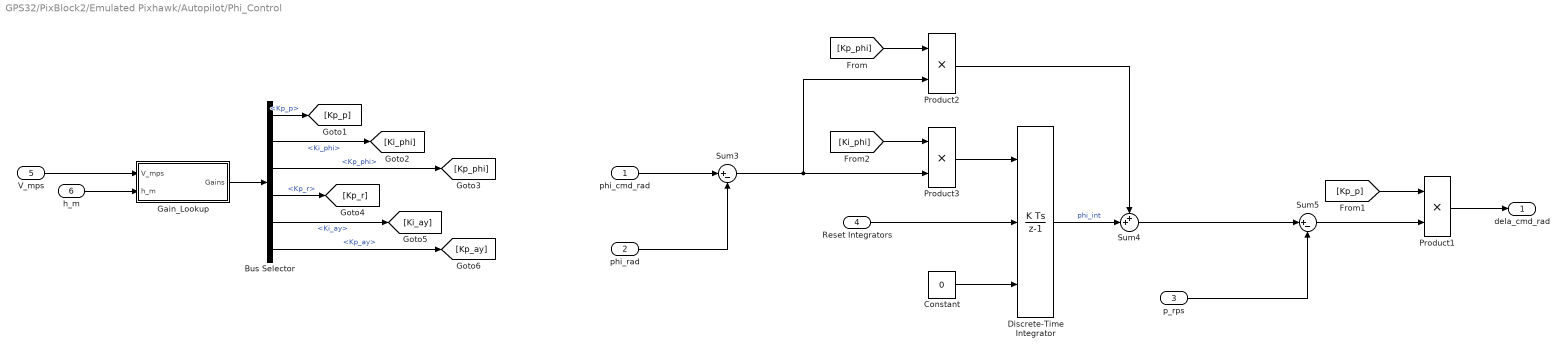
== system GPS32/PixBlock2/Emulated Pixhawk/Autopilot/Phi_Control ==
  phi_cmd_rad : Inport
  phi_rad : Inport  Port=2
  p_rps : Inport  Port=3
  Reset Integrators : Inport  Port=4
  V_mps : Inport  Port=5
  h_m : Inport  Port=6
  Bus Selector : BusSelector  OutputSignals=Kp_p,Ki_phi,Kp_phi,Kp_r,Ki_ay,Kp_ay
  Constant : Constant  Value=0  OutDataTypeStr=single
  Discrete-Time Integrator : DiscreteIntegrator  ExternalReset=level  InitialConditionSource=external  SampleTime=-1  OutDataTypeStr=single  ICPrevOutput=DiscIntNeverNeededParam  ICPrevScaledInput=DiscIntNeverNeededParam
  Gain_Lookup : Subsystem
  Product1 : Product
  Product2 : Product
  Product3 : Product
  Sum3 : Sum  Inputs=|+-
  Sum4 : Sum  Inputs=++|
  Sum5 : Sum  Inputs=|+-
  dela_cmd_rad : Outport
  wires:
  phi_cmd_rad/1 -> Sum3/1
  Reset Integrators/1 -> Discrete-Time Integrator/2
  p_rps/1 -> Sum5/2
  phi_rad/1 -> Sum3/2
  Product2/1 -> Sum4/1
  Sum3/1 -> Product3/2, Product2/2
  Constant/1 -> Discrete-Time Integrator/3
  Sum5/1 -> Product1/2
  [Ki_phi] -> Product3/1
  Product1/1 -> dela_cmd_rad/1
  [Kp_p] -> Product1/1
  [Kp_phi] -> Product2/1
  Discrete-Time Integrator/1 -> Sum4/2  "phi_int"
  Sum4/1 -> Sum5/1
  Product3/1 -> Discrete-Time Integrator/1
  h_m/1 -> Gain_Lookup/2(h_m)
  Bus Selector/6 -> [Kp_ay]  "<Kp_ay>"
  Bus Selector/5 -> [Ki_ay]  "<Ki_ay>"
  Bus Selector/2 -> [Ki_phi]  "<Ki_phi>"
  Bus Selector/1 -> [Kp_p]  "<Kp_p>"
  V_mps/1 -> Gain_Lookup/1(V_mps)
  Bus Selector/4 -> [Kp_r]  "<Kp_r>"
  Gain_Lookup/1(Gains) -> Bus Selector/1
  Bus Selector/3 -> [Kp_phi]  "<Kp_phi>"

== system GPS32/PixBlock2/Emulated Pixhawk/Fin Allocation/control_allocation ==
  fin_cmd : Inport
  Constant7 : Constant  Value=HIL_Data.FDM.Tr4r3  OutDataTypeStr=single
  Product : Product  Multiplication=Matrix(*)
  siB_cmd : Outport  VectorParamsAs1DForOutWhenUnconnected=off
  wires:
  Constant7/1 -> Product/1
  fin_cmd/1 -> Product/2
  Product/1 -> siB_cmd/1  "siB_cmd"

== system GPS32/PixBlock2/Emulated Pixhawk/Servo Commands/100Hz Progress ==
  Delay : Delay  DelayLength=1
  GreaterThan : RelationalOperator  Operator=>  OutDataTypeStr=boolean  RndMeth=Simplest
  RST : Outport
  wires:
  GreaterThan/1 -> RST/1
  Delay/1 -> GreaterThan/2
  [Heartbeat] -> Delay/1, GreaterThan/1

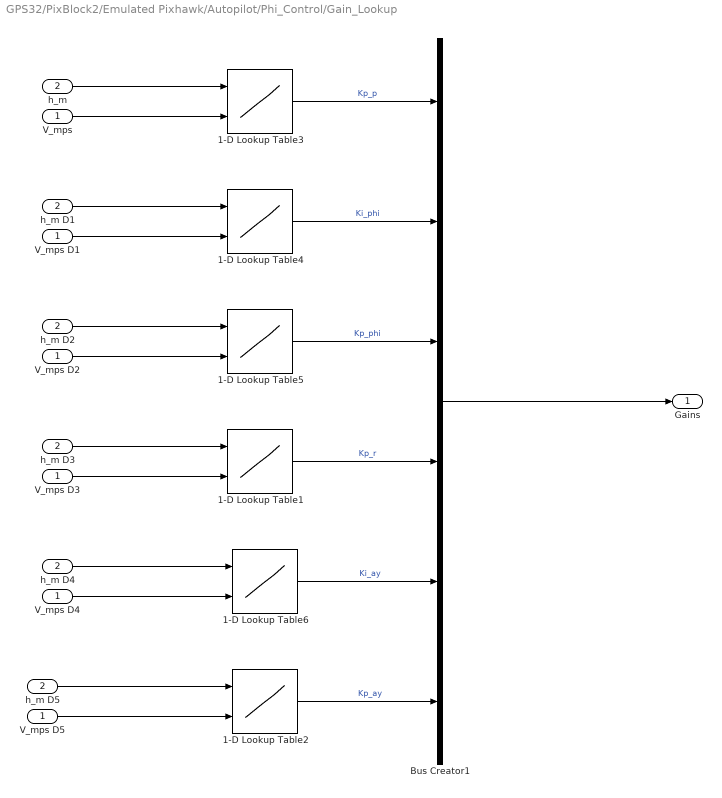
== system GPS32/PixBlock2/Emulated Pixhawk/Autopilot/Phi_Control/Gain_Lookup ==
  V_mps : Inport
  h_m : Inport  Port=2
  1-D Lookup Table1 : Lookup_n-D  BreakpointsForDimension1=Autopilot.Ay.h_bkpts_m  BreakpointsForDimension2=Autopilot.Ay.V_bkpts_mps  Table=Autopilot.Ay.Kp_r_vec  ExtrapMethod=Clip  UseLastTableValue=on  InternalRulePriority=Speed  RndMeth=Simplest  InputSameDT=on
      settings: InputPortMap=u0,u1
      settings: AttributesFormatString=|
      | %<Table>
      | %<BreakpointsForDimension1>
      | %<BreakpointsForDimension2>
  1-D Lookup Table2 : Lookup_n-D  BreakpointsForDimension1=Autopilot.Ay.h_bkpts_m  BreakpointsForDimension2=Autopilot.Ay.V_bkpts_mps  Table=Autopilot.Ay.Kp_ay_vec  ExtrapMethod=Clip  UseLastTableValue=on  InternalRulePriority=Speed  RndMeth=Simplest  InputSameDT=on
      settings: InputPortMap=u0,u1
      settings: AttributesFormatString=|
      | %<Table>
      | %<BreakpointsForDimension1>
      | %<BreakpointsForDimension2>
  1-D Lookup Table3 : Lookup_n-D  BreakpointsForDimension1=Autopilot.Phi.h_bkpts_m  BreakpointsForDimension2=Autopilot.Phi.V_bkpts_mps  Table=Autopilot.Phi.Kp_p_vec  ExtrapMethod=Clip  UseLastTableValue=on  InternalRulePriority=Speed  RndMeth=Simplest  InputSameDT=on
      settings: InputPortMap=u0,u1
      settings: AttributesFormatString=|
      | %<Table>
      | %<BreakpointsForDimension1>
      | %<BreakpointsForDimension2>
  1-D Lookup Table4 : Lookup_n-D  BreakpointsForDimension1=Autopilot.Phi.h_bkpts_m  BreakpointsForDimension2=Autopilot.Phi.V_bkpts_mps  Table=Autopilot.Phi.Ki_phi_vec  ExtrapMethod=Clip  UseLastTableValue=on  InternalRulePriority=Speed  RndMeth=Simplest  InputSameDT=on
      settings: InputPortMap=u0,u1
      settings: AttributesFormatString=|
      | %<Table>
      | %<BreakpointsForDimension1>
      | %<BreakpointsForDimension2>
  1-D Lookup Table5 : Lookup_n-D  BreakpointsForDimension1=Autopilot.Phi.h_bkpts_m  BreakpointsForDimension2=Autopilot.Phi.V_bkpts_mps  Table=Autopilot.Phi.Kp_phi_vec  ExtrapMethod=Clip  UseLastTableValue=on  InternalRulePriority=Speed  RndMeth=Simplest  InputSameDT=on
      settings: InputPortMap=u0,u1
      settings: AttributesFormatString=|
      | %<Table>
      | %<BreakpointsForDimension1>
      | %<BreakpointsForDimension2>
  1-D Lookup Table6 : Lookup_n-D  BreakpointsForDimension1=Autopilot.Ay.h_bkpts_m  BreakpointsForDimension2=Autopilot.Ay.V_bkpts_mps  Table=Autopilot.Ay.Ki_ay_vec  ExtrapMethod=Clip  UseLastTableValue=on  InternalRulePriority=Speed  RndMeth=Simplest  InputSameDT=on
      settings: InputPortMap=u0,u1
      settings: AttributesFormatString=|
      | %<Table>
      | %<BreakpointsForDimension1>
      | %<BreakpointsForDimension2>
  Bus Creator1 : BusCreator  Inputs=6
  V_mps D{1..5} (5 alike) : InportShadow
  h_m D{1..5} (5 alike) : InportShadow  Port=2
  Gains : Outport
  wires:
  h_m/1 -> 1-D Lookup Table3/1
  Bus Creator1/1 -> Gains/1
  1-D Lookup Table5/1 -> Bus Creator1/3  "Kp_phi"
  1-D Lookup Table4/1 -> Bus Creator1/2  "Ki_phi"
  1-D Lookup Table3/1 -> Bus Creator1/1  "Kp_p"
  V_mps/1 -> 1-D Lookup Table3/2
  h_m D1/1 -> 1-D Lookup Table4/1
  V_mps D1/1 -> 1-D Lookup Table4/2
  h_m D2/1 -> 1-D Lookup Table5/1
  V_mps D2/1 -> 1-D Lookup Table5/2
  1-D Lookup Table2/1 -> Bus Creator1/6  "Kp_ay"
  1-D Lookup Table6/1 -> Bus Creator1/5  "Ki_ay"
  1-D Lookup Table1/1 -> Bus Creator1/4  "Kp_r"
  h_m D3/1 -> 1-D Lookup Table1/1
  V_mps D3/1 -> 1-D Lookup Table1/2
  h_m D4/1 -> 1-D Lookup Table6/1
  V_mps D4/1 -> 1-D Lookup Table6/2
  h_m D5/1 -> 1-D Lookup Table2/1
  V_mps D5/1 -> 1-D Lookup Table2/2

== matlab function GPS32/MATLAB Function ==
  data: vx input; y output; vy input; vz input
function y = fcn(vx,vy,vz)

y = double(norm([vx vy vz]));
end

== matlab function GPS32/PX4 SD Card Logger3/SDCard_logger ==
  data: en input boolean; data input; logname parameter uint8; cacheflag parameter boolean; numRecs parameter uint32
%% PX4 SD Card Logger
% Note: All data needs to be of the same type (e.g. double)
% Header information format:
%           String "MWLOG"
%           Time/Date 4 bytes (time())
%           Number of Signals per record Logged 1 byte (256 max)
%           Data Type of Signals Logged  1 byte (1-10)
%           Number of bytes per record 2 bytes (65535 max)
% This does NOT include the number of data sets logged.
% i.e. The Reader is responsible for reading until EOF.
% Steve Kuznicki
% Copyright 2018 The MathWorks, Inc.

function SDCard_logger(en, data, logname, cacheflag, numRecs)

persistent fp isflushed isopen count  elem_size vect_size datastore timestore count_prev

if coder.target('Rtw')
    
    coder.cinclude('<stdio.h>');
    coder.cinclude('<time.h>');
    
    if coder.target('Rtw')
        coder.cinclude('<drivers/drv_hrt.h>');
    end
    
    if coder.target('Rtw')
        timestamp=coder.opaque('uint64_t');
        timestamp=coder.ceval('hrt_absolute_time');
    else
        timestamp = uint64(0);
    end
    
    if isempty(count)
        count = uint32(0);
        count_prev=count;
        fp = coder.opaque('FILE*', 'NULL');
        isflushed = false;
        if cacheflag == true
            datastore = zeros(numRecs*uint32(coder.const(numel(data))), 1, 'like', data);
            timestore=uint64(zeros(numRecs, 1));
        end
        
        [elsize, eltype] = get_elem_size(data);
        elem_size = coder.const(uint16(elsize));
        elem_type = coder.const(uint8(eltype));
        vect_size = coder.const(uint8(numel(data)));
        coder.ceval('printf',['OPENING file %s vect_size %d elem_size %d numRecs %d %c' uint8(0)], ...
            [logname,'.bin', int8(0)], uint32(vect_size), uint32(elem_size), uint32(numRecs), uint8(10));
        fp = coder.ceval('fopen', [logname,'.bin', int8(0)], ['wb', int8(0)]);
        isopen = true;
        
        % Write header information here
        % header token + version
        mlStrVer = 'MWLOG';
        coder.ceval('fwrite', coder.rref(mlStrVer), uint32(1), length(mlStrVer), fp);
        % date/time
        tm = uint32(0);
        tmptr = uint32(0);
        tm = coder.ceval('time',coder.wref(tmptr));
        coder.ceval('fwrite', coder.rref(tm), uint32(4), uint32(1), fp);
        % number of elements in each record
        coder.ceval('fwrite', coder.rref(vect_size), uint32(1), uint32(1), fp);
        % data type of the elements
        coder.ceval('fwrite', coder.rref(elem_type), uint32(1), uint32(1), fp);
        % size of each record in bytes
        recSize = elem_size * uint16(vect_size);
        coder.ceval('fwrite', coder.rref(recSize), uint32(2), uint32(1), fp);
    end
    
    
    if (en && (count < numRecs))
        
        if isopen == false
            % open file in append mode
            fp = coder.ceval('fopen', [logname,'.bin', int8(0)], ['ab', int8(0)]);
            isflushed = false;
            isopen = true;
            count_prev=count;
        end
        
        % cache data in memory or use fwrite
        if cacheflag == true
            addr = (count*uint32(vect_size))+1;
            for idx = 1:vect_size
                datastore(addr) = data(idx);
                addr = addr + 1;
            end
            timestore(count+uint32(1))=uint64(timestamp);
        else
            coder.ceval('fwrite', coder.rref(data), elem_size, vect_size, fp);
            if coder.target('Rtw')
                coder.ceval('fwrite', coder.rref(timestamp), uint32(8), uint32(1), fp);
            end
        end
        count = count + uint32(1);
        
    else
        if isopen == true
            if ~isflushed
                coder.ceval('printf',['CLOSING file. count = %d %c' uint8(0)], uint32(count), uint8(10));
                if cacheflag
                    for idx=count_prev+1:count
                        for idx2=(idx-1)*double(vect_size)+1:(idx-1)*double(vect_size)+double(vect_size)
                            coder.ceval('fwrite', coder.rref(datastore(idx2)), elem_size, uint32(1), fp);
                        end
                        coder.ceval('fwrite', coder.rref(timestore(idx)), uint32(8), uint32(1), fp);
                    end
                end
                coder.ceval('fflush', fp);
                isflushed = true;
            end
            coder.ceval('fclose', fp);
        end
        isopen = false;
    end
end

% return the size of the element in bytes
    function [elem_size, dtype] = get_elem_size(data)
        switch(class(data))
            case 'double'
                elem_size = 8;
                dtype = 1;
            case 'single'
                elem_size = 4;
                dtype = 2;
            case 'int32'
                elem_size = 4;
                dtype = 3;
            case 'uint32'
                elem_size = 4;
                dtype = 4;
            case 'int16'
                elem_size = 2;
                dtype = 5;
            case 'uint16'
                elem_size = 2;
                dtype = 6;
            case 'int8'
                elem_size = 1;
                dtype = 7;
            case 'uint8'
                elem_size = 1;
                dtype = 8;
            case 'logical'
                elem_size = 1;
                dtype = 9;
            case 'embedded.fi'
                nt = numerictype(data);
                elem_size = 2^ceil(log2(ceil(nt.WordLength / 8)));
                dtype = 10;
        end
        if ~isreal(data)
            elem_size = elem_size*2;
        end
        
        elem_size = uint16(elem_size);
        dtype = uint8(dtype);
    end
end
